simulink model "assi2_q2_simu"  (R2022a)
settings: Solver=VariableStepAuto  StartTime=0.0  StopTime=10e3  RelTol=1e-3
undefined symbols (not defined in the file): m, n
settings Model: Creator=Yinhao  LastModifiedBy=Yinhao

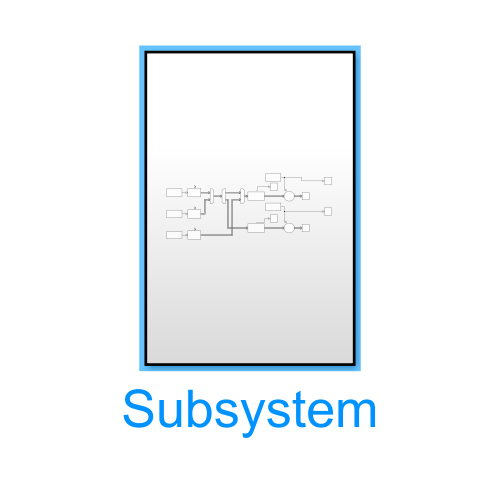
[thumbnail: Simulink's stored preview of the top-level diagram]
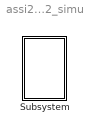
== system assi2_q2_simu ==
  Subsystem : Subsystem

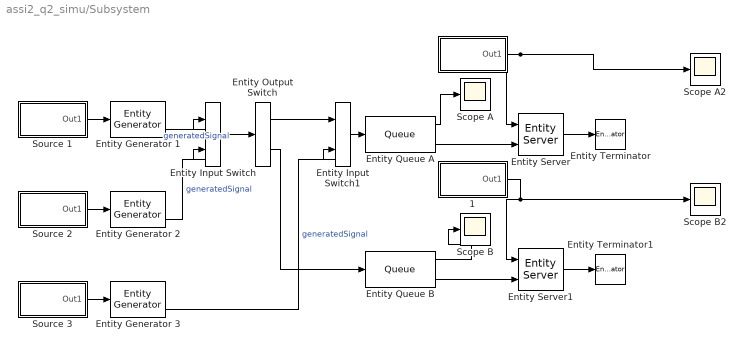
== system assi2_q2_simu/Subsystem ==
  " " : Subsystem  mask(Exponential Random Number){mean=1/14, seed=1414}
      mask prompts: seed "Random Seed"
      mask help: This block generate a random number with exponential distribution.
      mask Display: disp(['mean=' num2str(mean,2)],"texmode","on");
  " 1" : Subsystem  mask(Exponential Random Number){mean=1/12, seed=1212}
      mask prompts: seed "Random Seed"
      mask help: This block generate a random number with exponential distribution.
      mask Display: disp(['mean=' num2str(mean,2)],"texmode","on");
  Entity Input Switch : EntityInputSwitch  InputPortMessageModes=m,m  OutputPortMessageModes=m
  Entity Input Switch1 : EntityInputSwitch  InputPortMessageModes=m,m  OutputPortMessageModes=m
  Entity Output Switch : EntityOutputSwitch  InputPortMessageModes=m  OutputPortMessageModes=m,m  SwitchingCriterion=From attribute  SwitchAttributeName=path
  Entity Generator 1 : EntityGenerator  OutputPortMessageModes=n,m  TimeSource=Signal port  GenerateAction=|  AttributeName=path  AttributeInitialValue=0  NumberEntitiesDeparted=on  EntityType=Structured  EntityTypeName=Entity
      | pathIndex = rand();
      | if(rand<=0.25)
      |     entity.path = 1;
      | else
      |     entity.path = 2;
      | end
      settings: InputPortMap=u1  OutputPortMap=o0,o3
  Entity Generator 2 : EntityGenerator  OutputPortMessageModes=n,m  TimeSource=Signal port  GenerateAction=|  AttributeName=path  AttributeInitialValue=0  NumberEntitiesDeparted=on  EntityType=Structured  EntityTypeName=Entity
      | pathIndex = rand();
      | if(rand<=0.25)
      |     entity.path = 1;
      | else
      |     entity.path = 2;
      | end
      settings: InputPortMap=u1  OutputPortMap=o0,o3
  Entity Generator 3 : EntityGenerator  OutputPortMessageModes=n,m  TimeSource=Signal port  GenerateAction=entity.path = 0;  AttributeName=path  NumberEntitiesDeparted=on  EntityType=Structured  EntityTypeName=Entity
      settings: InputPortMap=u1  OutputPortMap=o0,o3
  Entity Queue A : Queue  InputPortMessageModes=m  OutputPortMessageModes=n,m  Capacity=inf  AverageWait=on
      settings: OutputPortMap=o2,o5
  Entity Queue B : Queue  InputPortMessageModes=m  OutputPortMessageModes=n,m  Capacity=inf  AverageWait=on
      settings: OutputPortMap=o2,o5
  Entity Server : EntityServer  InputPortMessageModes=n,m  OutputPortMessageModes=m  Capacity=1  ServiceTimeSource=Signal port  ServiceTimeValue=2/3
      settings: InputPortMap=u0,u2
  Entity Server1 : EntityServer  InputPortMessageModes=n,m  OutputPortMessageModes=m  Capacity=1  ServiceTimeSource=Signal port  ServiceTimeValue=2/3
      settings: InputPortMap=u0,u2
  Entity Terminator : EntityTerminator  InputPortMessageModes=m
  Entity Terminator1 : EntityTerminator  InputPortMessageModes=m
  Scope A : Scope
  Scope A2 : Scope
  Scope B : Scope
  Scope B2 : Scope
  Source 1 : Subsystem  mask(Exponential Random Number){mean=1/9, seed=999}
      mask prompts: seed "Random Seed"
      mask help: This block generate a random number with exponential distribution.
      mask Display: disp(['mean=' num2str(mean,2)],"texmode","on");
  Source 2 : Subsystem  mask(Exponential Random Number){mean=1/3, seed=333}
      mask prompts: seed "Random Seed"
      mask help: This block generate a random number with exponential distribution.
      mask Display: disp(['mean=' num2str(mean,2)],"texmode","on");
  Source 3 : Subsystem  mask(Exponential Random Number){mean=1/4, seed=444}
      mask prompts: seed "Random Seed"
      mask help: This block generate a random number with exponential distribution.
      mask Display: disp(['mean=' num2str(mean,2)],"texmode","on");
  wires:
  Entity Queue A/2 -> Entity Server/2
  Entity Queue A/1 -> Scope A/1
  Entity Server/1 -> Entity Terminator/1
  Source 1/1(Out1) -> Entity Generator 1/1
  Source 2/1(Out1) -> Entity Generator 2/1
  Source 3/1(Out1) -> Entity Generator 3/1
  Entity Generator 1/2 -> Entity Input Switch/1  "generatedSignal"
  Entity Generator 2/2 -> Entity Input Switch/2  "generatedSignal"
  Entity Input Switch/1 -> Entity Output Switch/1
  Entity Generator 3/2 -> Entity Input Switch1/2  "generatedSignal"
  Entity Output Switch/1 -> Entity Input Switch1/1
  Entity Input Switch1/1 -> Entity Queue A/1
  Entity Output Switch/2 -> Entity Queue B/1
  Entity Server1/1 -> Entity Terminator1/1
  Entity Queue B/1 -> Scope B/1
  Entity Queue B/2 -> Entity Server1/2
  " 1"/1(Out1) -> Scope B2/1, Entity Server1/1
  " "/1(Out1) -> Entity Server/1, Scope A2/1

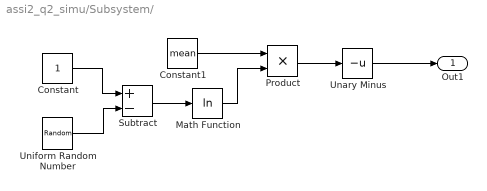
== system assi2_q2_simu/Subsystem/  ==
  Constant : Constant
  Constant1 : Constant  Value=mean
  Math Function : Math  Operator=log  SignedPower=on
  Product : Product  RndMeth=Zero
  Subtract : Sum  Inputs=+-
  Unary Minus : UnaryMinus
  Uniform Random Number : UniformRandomNumber  Minimum=0  Seed=seed
  Out1 : Outport
  wires:
  Subtract/1 -> Math Function/1
  Math Function/1 -> Product/2
  Unary Minus/1 -> Out1/1
  Product/1 -> Unary Minus/1
  Constant/1 -> Subtract/1
  Uniform Random Number/1 -> Subtract/2
  Constant1/1 -> Product/1

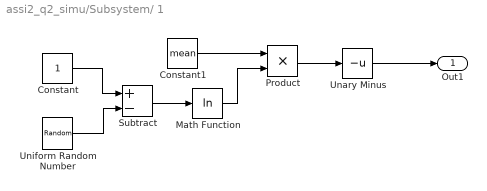
== system assi2_q2_simu/Subsystem/ 1 ==
  Constant : Constant
  Constant1 : Constant  Value=mean
  Math Function : Math  Operator=log  SignedPower=on
  Product : Product  RndMeth=Zero
  Subtract : Sum  Inputs=+-
  Unary Minus : UnaryMinus
  Uniform Random Number : UniformRandomNumber  Minimum=0  Seed=seed
  Out1 : Outport
  wires:
  Subtract/1 -> Math Function/1
  Math Function/1 -> Product/2
  Unary Minus/1 -> Out1/1
  Product/1 -> Unary Minus/1
  Constant/1 -> Subtract/1
  Uniform Random Number/1 -> Subtract/2
  Constant1/1 -> Product/1

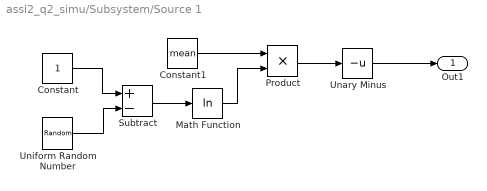
== system assi2_q2_simu/Subsystem/Source 1 ==
  Constant : Constant
  Constant1 : Constant  Value=mean
  Math Function : Math  Operator=log  SignedPower=on
  Product : Product  RndMeth=Zero
  Subtract : Sum  Inputs=+-
  Unary Minus : UnaryMinus
  Uniform Random Number : UniformRandomNumber  Minimum=0  Seed=seed
  Out1 : Outport
  wires:
  Subtract/1 -> Math Function/1
  Math Function/1 -> Product/2
  Unary Minus/1 -> Out1/1
  Product/1 -> Unary Minus/1
  Constant/1 -> Subtract/1
  Uniform Random Number/1 -> Subtract/2
  Constant1/1 -> Product/1

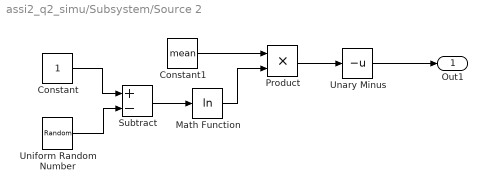
== system assi2_q2_simu/Subsystem/Source 2 ==
  Constant : Constant
  Constant1 : Constant  Value=mean
  Math Function : Math  Operator=log  SignedPower=on
  Product : Product  RndMeth=Zero
  Subtract : Sum  Inputs=+-
  Unary Minus : UnaryMinus
  Uniform Random Number : UniformRandomNumber  Minimum=0  Seed=seed
  Out1 : Outport
  wires:
  Subtract/1 -> Math Function/1
  Math Function/1 -> Product/2
  Unary Minus/1 -> Out1/1
  Product/1 -> Unary Minus/1
  Constant/1 -> Subtract/1
  Uniform Random Number/1 -> Subtract/2
  Constant1/1 -> Product/1

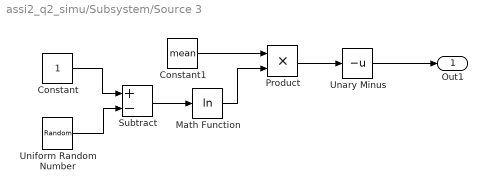
== system assi2_q2_simu/Subsystem/Source 3 ==
  Constant : Constant
  Constant1 : Constant  Value=mean
  Math Function : Math  Operator=log  SignedPower=on
  Product : Product  RndMeth=Zero
  Subtract : Sum  Inputs=+-
  Unary Minus : UnaryMinus
  Uniform Random Number : UniformRandomNumber  Minimum=0  Seed=seed
  Out1 : Outport
  wires:
  Subtract/1 -> Math Function/1
  Math Function/1 -> Product/2
  Unary Minus/1 -> Out1/1
  Product/1 -> Unary Minus/1
  Constant/1 -> Subtract/1
  Uniform Random Number/1 -> Subtract/2
  Constant1/1 -> Product/1
